simulink model "ClosedFormIK_Simul"  (R2024b)
settings: Solver=VariableStepAuto  StartTime=0.0  StopTime=inf  RelTol=1e-3
libraries: vrlib x7, simulink x3, ClosedFormIK_Lib x1
settings Model: Creator=pepev  LastModifiedBy=pepev

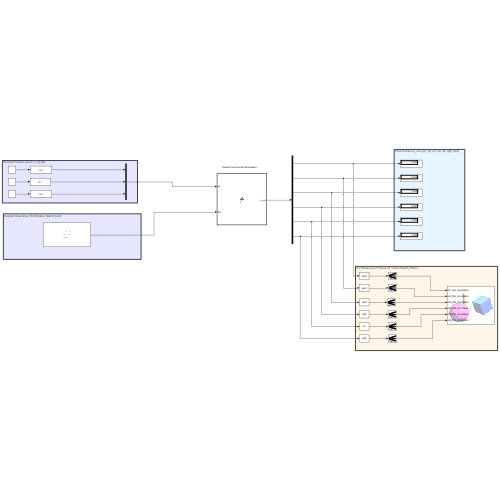
[thumbnail: Simulink's stored preview of the top-level diagram]
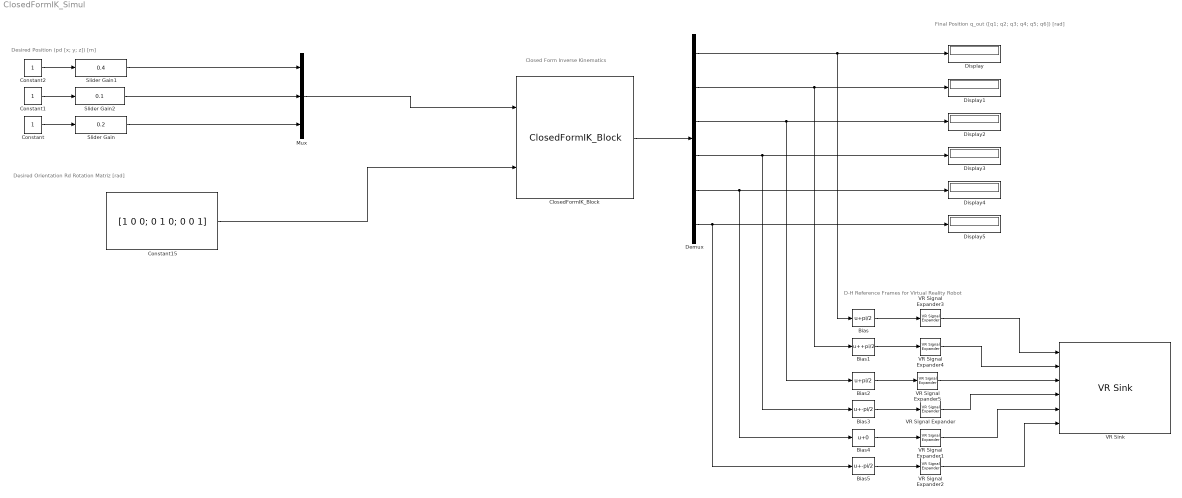
== system ClosedFormIK_Simul ==
  note: Closed Form Inverse Kinematics
  note: Final Position q_out ([q1; q2; q3; q4; q5; q6]) [rad]
  note: Desired Orientation Rd Rotation Matriz [rad]
  note: Desired Position (pd [x; y; z]) [m]
  note: D-H Reference Frames for Virtual Reality Robot
  Bias : Bias  Bias=pi/2  SaturateOnIntegerOverflow=off
  Bias1 : Bias  Bias=+pi/2  SaturateOnIntegerOverflow=off
  Bias2 : Bias  Bias=pi/2  SaturateOnIntegerOverflow=off
  Bias3 : Bias  Bias=-pi/2  SaturateOnIntegerOverflow=off
  Bias4 : Bias  SaturateOnIntegerOverflow=off
  Bias5 : Bias  Bias=-pi/2  SaturateOnIntegerOverflow=off
  ClosedFormIK_Block : ClosedFormIK_Lib/ClosedFormIK_Block  SystemSampleTime=-1  VariantActivationTime=update diagram  AllowFlexibleInterface=on  Latency=0  AutoFrameSizeCalculation=off
  Constant : Constant
  Constant1 : Constant
  Constant15 : Constant  Value=[1 0 0; 0 1 0; 0 0 1]
  Constant2 : Constant
  Demux : Demux  Outputs=6
  Display{,1..5} (6 alike) : Display
  Mux : Mux  Inputs=3
  Slider Gain : simulink/Math Operations/Slider Gain  gain=0.2  low=-1  high=1
  Slider Gain1 : simulink/Math Operations/Slider Gain  gain=0.4  low=-3.14  high=3.14
  Slider Gain2 : simulink/Math Operations/Slider Gain  gain=0.1  low=-3.14  high=3.14
  VR Signal Expander{,1..5} (6 alike) : vrlib/VR Signal Expander  outwidth=4  outidx=[4]
  VR Sink : vrlib/VR Sink  InstantiateOnLoad=on  SampleTime=-1  ViewEnable=on  RemoteChange=off  RemoteView=off  FieldsWritten=Jt1_DH_dv.rotation.4.1.1.double#Jt2_DH_dv.rotation.4.1.1.double#Jt3_DH_dv.rotation.4.1.1.double#Jt4_DH_dv.rotation.4.1.1.double#Jt5_DH_dv.rotation.4.1.1.double#Jt6_DH_dv.rotation.4.1.1.double  WorldFileName=vrrobot.wrl  WorldDescription=D-H Reference Frames for Virtual Reality Robot  AutoView=on  VideoDimensions=[]  AllowVariableSize=off
  wires:
  Constant15/1 -> ClosedFormIK_Block/2
  VR Signal Expander1/1 -> VR Sink/5
  Bias4/1 -> VR Signal Expander1/1
  Slider Gain2/1 -> Mux/2
  Slider Gain/1 -> Mux/3
  Mux/1 -> ClosedFormIK_Block/1
  Bias1/1 -> VR Signal Expander4/1
  Demux/5 -> Display4/1, Bias4/1
  VR Signal Expander5/1 -> VR Sink/3
  VR Signal Expander3/1 -> VR Sink/1
  ClosedFormIK_Block/1 -> Demux/1
  Constant/1 -> Slider Gain/1
  Bias5/1 -> VR Signal Expander2/1
  Bias2/1 -> VR Signal Expander5/1
  VR Signal Expander4/1 -> VR Sink/2
  Demux/3 -> Bias2/1, Display2/1
  VR Signal Expander2/1 -> VR Sink/6
  VR Signal Expander/1 -> VR Sink/4
  Slider Gain1/1 -> Mux/1
  Bias/1 -> VR Signal Expander3/1
  Constant2/1 -> Slider Gain1/1
  Demux/2 -> Bias1/1, Display1/1
  Bias3/1 -> VR Signal Expander/1
  Demux/1 -> Bias/1, Display/1
  Demux/4 -> Bias3/1, Display3/1
  Demux/6 -> Bias5/1, Display5/1
  Constant1/1 -> Slider Gain2/1
